simulink model "forward_torque"  (R2020a)
settings: Solver=VariableStepAuto  StartTime=0.0  StopTime=10.0  RelTol=1e-3
undefined symbols (not defined in the file): p560
libraries: roblocks x4
settings Model: Creator=yuan_  LastModifiedBy=yuan_

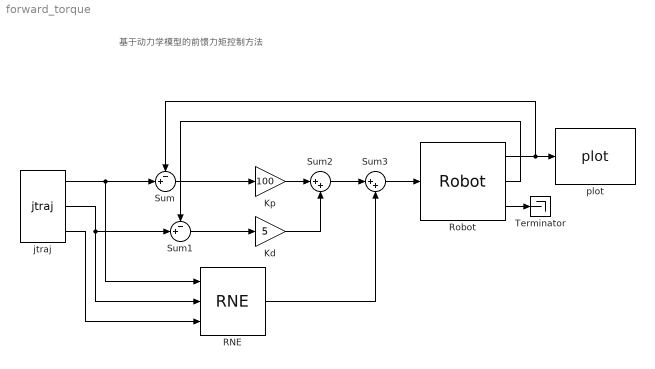
== system forward_torque ==
  note: 基于动力学模型的前馈力矩控制方法
  Kd : Gain  Gain=5  SaturateOnIntegerOverflow=on  OutDataTypeStr=Inherit: Same as input  ParamDataTypeStr=Inherit: Same as input
  Kp : Gain  Gain=100  SaturateOnIntegerOverflow=on  OutDataTypeStr=Inherit: Same as input  ParamDataTypeStr=Inherit: Same as input
  RNE : roblocks/Arm/RNE  robot=p560.nofriction()  grav=[0 0 9.81]
  Robot : roblocks/Arm/Robot  robot=p560.nofriction  q0=[0 0 0 0 0 0]
  Sum : Sum  Inputs=-+|  InputSameDT=on  SaturateOnIntegerOverflow=on  OutDataTypeStr=Inherit: Same as first input
  Sum1 : Sum  Inputs=-+|  InputSameDT=on  SaturateOnIntegerOverflow=on  OutDataTypeStr=Inherit: Same as first input
  Sum2 : Sum  Inputs=|++  InputSameDT=on  SaturateOnIntegerOverflow=on  OutDataTypeStr=Inherit: Same as first input
  Sum3 : Sum  Inputs=|++  InputSameDT=on  SaturateOnIntegerOverflow=on  OutDataTypeStr=Inherit: Same as first input
  Terminator : Terminator
  jtraj : roblocks/Toolbox/jtraj  q0=[0 0 0 0 0 0]  qf=[pi/4 pi/2 -pi/2 0 0 0]  tmax=5  ts=0.02
  plot : roblocks/Arm/plot  robot=p560  fps=10  holdplot=on
  wires:
  Robot/3 -> Terminator/1
  Sum2/1 -> Sum3/1
  Robot/2 -> Sum1/1
  jtraj/2 -> RNE/2, Sum1/2
  Robot/1 -> plot/1, Sum/1
  Kp/1 -> Sum2/1
  Sum1/1 -> Kd/1
  RNE/1 -> Sum3/2
  Sum/1 -> Kp/1
  jtraj/1 -> RNE/1, Sum/2
  Sum3/1 -> Robot/1
  jtraj/3 -> RNE/3
  Kd/1 -> Sum2/2
